simulink library "lic"  (R2021b)
settings: Solver=VariableStepAuto  StartTime=0.0  StopTime=10.0  RelTol=1e-3
undefined symbols (not defined in the file or in its folder): C_TICK_TIME_S, ENUM_LANEQUALITY_HIGH, ENUM_LANEQUALITY_MEDIUM, ENUM_LFCSTATE_DEGRADED, FALSE, KAPP_VehicleWidth_m, KLIC_C0CrossingThr_m, KLIC_C1Max4Act_rad, KLIC_C2Max4Act_rat, KLIC_C2Max4Disable_rat, KLIC_C2Max4DisableThr_s, KLIC_CalDefaultTLC_s, KLIC_CalTLCMax_s, KLIC_CalTLCMin_s, KLIC_DefaultLaneWidth_m, KLIC_Lane4ActThr_s, KLIC_LANEQUALITY_rat, KLIC_LANEQUALITYHysis_rat, KLIC_LaneWidHoldOnTime_s, KLIC_LaneWidRampFinErrThres_m, KLIC_LaneWidRampFinTimeThres_s, KLIC_LaneWidRampInFalRt_mps, KLIC_LaneWidRampInRisRt_mps, KLIC_LaneWidRampOutFalRt_mps, KLIC_LaneWidRampOutRisRt_mps, KLIC_LaneWidthLowThr_m, KLIC_LaneWidthUpThr_m, KLIC_TLCTriggerThrHysis_s, MLIC_TLCThr4LKA_s, TRUE
libraries: adcu_lib x20, simulink x14
(part 2 of 3)

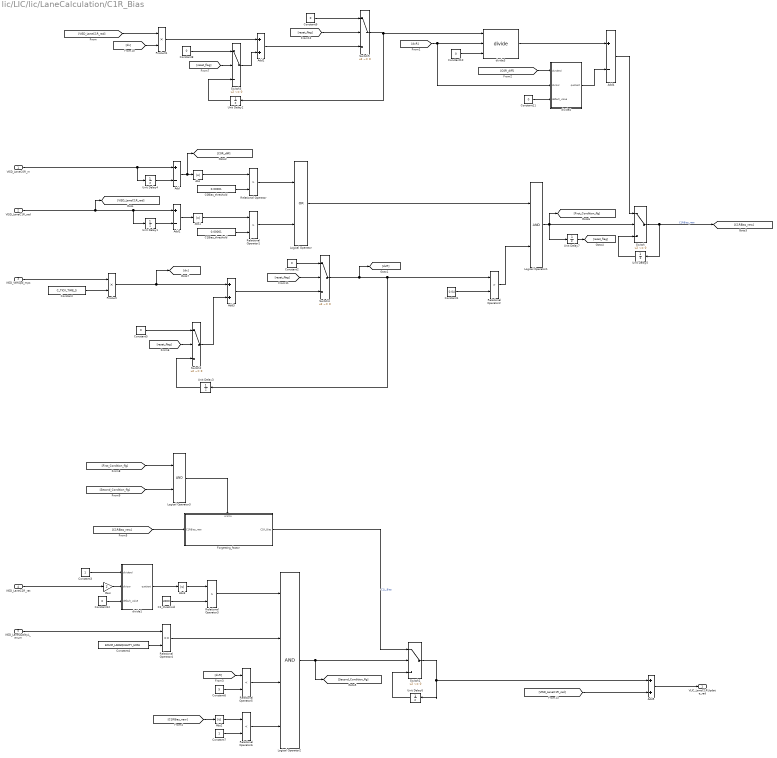
== system lic/LIC/lic/LaneCalculation/C1R_Bias ==
  VISD_LaneC0R_m : Inport
  VISD_LaneC1R_rad : Inport  Port=2
  VISD_VehSpd_mps : Inport  Port=3
  VISD_LaneC2R_rat : Inport  Port=4
  VISD_LaneQualityL_enum : Inport  Port=5
  Abs{,1..3} (4 alike) : Abs
  Add : Sum  Inputs=+-
  Add1 : Sum  Inputs=+-
  Add2 : Sum
  Add3 : Sum
  Add4 : Sum  Inputs=+-
  Add5 : Sum
  C0Bias_threshold : Constant  Value=0.00001  OutDataTypeStr=single
  C1Bias_threshold : Constant  Value=0.00001  OutDataTypeStr=single
  C2_threshold : Constant  Value=3000  OutDataTypeStr=single
  Constant : Constant  Value=C_TICK_TIME_S
  Constant1 : Constant  Value=0.04  OutDataTypeStr=single
  Constant{2,5,8..12} (7 alike) : Constant  Value=0  OutDataTypeStr=single
  Constant3 : Constant  OutDataTypeStr=single
  Constant4 : Constant  Value=ENUM_LANEQUALITY_HIGH
  Constant6 : Constant  Value=5  OutDataTypeStr=single
  Constant7 : Constant  OutDataTypeStr=single
  Forgetting_factor : Subsystem  TreatAsAtomicUnit=on
  Gain : Gain  Gain=2
  Logical Operator : Logic  Operator=OR  AllPortsSameDT=off  OutDataTypeStr=boolean
  Logical Operator1 : Logic  AllPortsSameDT=off  OutDataTypeStr=boolean
  Logical Operator2 : Logic  Inputs=4  AllPortsSameDT=off  OutDataTypeStr=boolean
  Logical Operator3 : Logic  AllPortsSameDT=off  OutDataTypeStr=boolean
  Product : Product
  Product1 : Product
  Relational Operator{,1..3} (4 alike) : RelationalOperator  Operator=>  OutDataTypeStr=boolean  RndMeth=Nearest
  Relational Operator4 : RelationalOperator  Operator===  OutDataTypeStr=boolean  RndMeth=Nearest
  Relational Operator5 : RelationalOperator  Operator=<  OutDataTypeStr=boolean  RndMeth=Nearest
  Relational Operator6 : RelationalOperator  Operator=<  OutDataTypeStr=boolean  RndMeth=Nearest
  Switch{,1..5} (6 alike) : Switch  Criteria=u2 ~= 0
  Unit Delay{1..7} (7 alike) : UnitDelay  SampleTime=-1  HasFrameUpgradeWarning=on
  divide1 : Subsystem  TreatAsAtomicUnit=on  RTWFcnName=divide_lib  RTWFileName=HCU_LIB  mask(divide){}
      mask help: Performs a division operation. If the divisor is found to be between -0.00001 and +0.00001 then a failsafe value is passed to the output.
      settings: RTWFcnNameOpts=User specified  RTWFileNameOpts=User specified
      mask Display: disp('Divide');
  divide3 : adcu_lib/divide
      settings: SourceProductName=ADAS Reusable Library
  divide4 : Subsystem  TreatAsAtomicUnit=on  RTWFcnName=divide_lib  RTWFileName=HCU_LIB  mask(divide){}
      mask help: Performs a division operation. If the divisor is found to be between -0.00001 and +0.00001 then a failsafe value is passed to the output.
      settings: RTWFcnNameOpts=User specified  RTWFileNameOpts=User specified
      mask Display: disp('Divide');
  VLIC_LaneC1RUpdate_rad : Outport
  wires:
  Add5/1 -> VLIC_LaneC1RUpdate_rad/1
  [VISD_LaneC1R_rad] -> Add5/2
  VISD_LaneC0R_m/1 -> Unit Delay4/1, Add/1
  Unit Delay4/1 -> Add/2
  VISD_LaneC1R_rad/1 -> [VISD_LaneC1R_rad], Unit Delay1/1, Add1/1
  Unit Delay1/1 -> Add1/2
  Add/1 -> [C0R_diff], Abs/1
  Add1/1 -> Abs1/1
  VISD_VehSpd_mps/1 -> Product/1
  Abs/1 -> Relational Operator/1
  C0Bias_threshold/1 -> Relational Operator/2
  Abs1/1 -> Relational Operator1/1
  C1Bias_threshold/1 -> Relational Operator1/2
  Add3/1 -> Switch4/3
  Constant1/1 -> Relational Operator2/2
  Relational Operator/1 -> Logical Operator/1
  Relational Operator1/1 -> Logical Operator/2
  Logical Operator/1 -> Logical Operator1/1
  Relational Operator2/1 -> Logical Operator1/2
  Logical Operator1/1 -> Switch/2, [First_Condition_flg], Unit Delay7/1
  [dx] -> Product1/2
  [VISD_LaneC1R_rad] -> Product1/1
  Product1/1 -> Add2/1
  Constant/1 -> Product/2
  Product/1 -> [dx], Add3/1
  [dxR] -> divide4/2(divisor), divide3/2
  divide3/1 -> Add4/1
  [C0R_diff] -> divide4/1(dividend)
  divide4/1(quotient) -> Add4/2
  Add4/1 -> Switch/1
  VISD_LaneC2R_rat/1 -> Gain/1
  divide1/1(quotient) -> Abs3/1
  C2_threshold/1 -> Relational Operator3/2
  VISD_LaneQualityL_enum/1 -> Relational Operator4/1
  Constant4/1 -> Relational Operator4/2
  Relational Operator3/1 -> Logical Operator2/1
  Relational Operator4/1 -> Logical Operator2/2
  [dxR] -> Relational Operator5/1
  Constant6/1 -> Relational Operator5/2
  Relational Operator5/1 -> Logical Operator2/3
  Relational Operator6/1 -> Logical Operator2/4
  Switch/1 -> Unit Delay5/1, [C1RBias_new]  "C1RBias_new"
  Switch1/1 -> Unit Delay6/1, Add5/1
  [C1RBias_new] -> Abs2/1
  Abs2/1 -> Relational Operator6/1
  Constant7/1 -> Relational Operator6/2
  Forgetting_factor/1(C1R_Bias) -> Switch1/1  "C1L_Bias"
  [C1RBias_new] -> Forgetting_factor/1(C1RBias_new)
  Unit Delay5/1 -> Switch/3
  Unit Delay6/1 -> Switch1/3
  Abs3/1 -> Relational Operator3/1
  Logical Operator2/1 -> [Second_Condition_flg], Switch1/2
  Switch2/1 -> Add3/2
  Constant5/1 -> Switch2/1
  [reset_flag] -> Switch2/2
  Constant8/1 -> Switch3/1
  [reset_flag] -> Switch3/2
  Switch3/1 -> Add2/2
  Unit Delay7/1 -> [reset_flag]
  Unit Delay2/1 -> Switch3/3
  Unit Delay3/1 -> Switch2/3
  [First_Condition_flg] -> Logical Operator3/1
  [Second_Condition_flg] -> Logical Operator3/2
  Logical Operator3/1 -> Forgetting_factor/Enable
  [reset_flag] -> Switch4/2
  Constant2/1 -> Switch4/1
  Switch4/1 -> [dxR], Unit Delay3/1, Relational Operator2/1
  Add2/1 -> Switch5/3
  [reset_flag] -> Switch5/2
  Constant9/1 -> Switch5/1
  Switch5/1 -> divide3/1, Unit Delay2/1
  Constant10/1 -> divide3/3
  Constant11/1 -> divide4/3(default_value)
  Constant3/1 -> divide1/1(dividend)
  Gain/1 -> divide1/2(divisor)
  Constant12/1 -> divide1/3(default_value)

== system lic/LIC/lic/LaneCalculation/GenerateLeftLane ==
  VISD_LaneC0L_m : Inport
  VLIC_EstLaneC0L_m : Inport  Port=2
  VISD_LaneC1L_rad : Inport  Port=3
  VLIC_EstLaneC1L_rad : Inport  Port=4
  VISD_LaneC2L_rat : Inport  Port=5
  VLIC_EstLaneC2L_rat : Inport  Port=6
  VISD_LaneC3L_rat : Inport  Port=7
  VLIC_EstLaneC3L_rat : Inport  Port=8
  VLIC_LeftLaneAvail_flg : Inport  Port=9
  Switch{3,12..14} (4 alike) : Switch  Criteria=u2 ~= 0
  VLIC_LaneC0L_m : Outport
  VLIC_LaneC1L_rad : Outport  Port=2
  VLIC_LaneC2L_rat : Outport  Port=3
  VLIC_LaneC3L_rat : Outport  Port=4
  wires:
  VLIC_EstLaneC0L_m/1 -> Switch3/3
  Switch12/1 -> VLIC_LaneC1L_rad/1  "VLIC_LaneC1L_rad"
  VLIC_EstLaneC1L_rad/1 -> Switch12/3
  VISD_LaneC1L_rad/1 -> Switch12/1
  Switch3/1 -> VLIC_LaneC0L_m/1  "VLIC_LaneC0L_m"
  Switch13/1 -> VLIC_LaneC2L_rat/1  "VLIC_LaneC2L_rat"
  VLIC_EstLaneC2L_rat/1 -> Switch13/3
  VISD_LaneC2L_rat/1 -> Switch13/1
  VLIC_LeftLaneAvail_flg/1 -> Switch14/2, Switch13/2, Switch12/2, Switch3/2
  VLIC_EstLaneC3L_rat/1 -> Switch14/3
  VISD_LaneC3L_rat/1 -> Switch14/1
  VISD_LaneC0L_m/1 -> Switch3/1
  Switch14/1 -> VLIC_LaneC3L_rat/1  "VLIC_LaneC3L_rat"

== system lic/LIC/lic/LaneCalculation/GenerateRightLane ==
  VISD_LaneC0R_m : Inport
  VLIC_EstLaneC0R_m : Inport  Port=2
  VISD_LaneC1R_rad : Inport  Port=3
  VLIC_EstLaneC1R_rad : Inport  Port=4
  VISD_LaneC2R_rat : Inport  Port=5
  VLIC_EstLaneC2R_rat : Inport  Port=6
  VISD_LaneC3R_rat : Inport  Port=7
  VLIC_EstLaneC3R_rat : Inport  Port=8
  VLIC_RightLaneAvail_flg : Inport  Port=9
  Switch{3,12..14} (4 alike) : Switch  Criteria=u2 ~= 0
  VLIC_LaneC0R_m : Outport
  VLIC_LaneC1R_rad : Outport  Port=2
  VLIC_LaneC2R_rat : Outport  Port=3
  VLIC_LaneC3R_rat : Outport  Port=4
  wires:
  VISD_LaneC0R_m/1 -> Switch3/1
  VISD_LaneC3R_rat/1 -> Switch14/1
  VLIC_EstLaneC3R_rat/1 -> Switch14/3
  Switch14/1 -> VLIC_LaneC3R_rat/1  "VLIC_LaneC3R_rat"
  VLIC_RightLaneAvail_flg/1 -> Switch3/2, Switch12/2, Switch13/2, Switch14/2
  VISD_LaneC2R_rat/1 -> Switch13/1
  VLIC_EstLaneC2R_rat/1 -> Switch13/3
  Switch13/1 -> VLIC_LaneC2R_rat/1  "VLIC_LaneC2R_rat"
  Switch3/1 -> VLIC_LaneC0R_m/1  "VLIC_LaneC0R_m"
  VISD_LaneC1R_rad/1 -> Switch12/1
  VLIC_EstLaneC1R_rad/1 -> Switch12/3
  Switch12/1 -> VLIC_LaneC1R_rad/1  "VLIC_LaneC1R_rad"
  VLIC_EstLaneC0R_m/1 -> Switch3/3

== system lic/LIC/lic/LaneCalculation/LR_Available ==
  VISD_LaneC0L_m : Inport
  VISD_LaneC0R_m : Inport  Port=2
  VISD_LaneC1L_rad : Inport  Port=3
  VISD_LaneC1R_rad : Inport  Port=4
  VISD_LaneC2L_rat : Inport  Port=5
  VISD_LaneC2R_rat : Inport  Port=6
  VISD_LaneC3L_rat : Inport  Port=7
  VISD_LaneC3R_rat : Inport  Port=8
  Enable : EnablePort  StatesWhenEnabling=reset
  Add{,1..3} (4 alike) : Sum
  Gain{,1..3} (4 alike) : Gain  Gain=0.5
  VLIC_RLCenterLineC0_m : Outport
  VLIC_RLCenterLineC1_rad : Outport  Port=2
  VLIC_RLCenterLineC2_rat : Outport  Port=3
  VLIC_RLCenterLineC3_rat : Outport  Port=4
  wires:
  VISD_LaneC0L_m/1 -> Add/1
  VISD_LaneC0R_m/1 -> Add/2
  Add/1 -> Gain/1
  Gain/1 -> VLIC_RLCenterLineC0_m/1  "VLIC_RLCenterLineC0_m"
  VISD_LaneC1L_rad/1 -> Add1/1
  VISD_LaneC1R_rad/1 -> Add1/2
  Add1/1 -> Gain1/1
  Add2/1 -> Gain2/1
  Gain1/1 -> VLIC_RLCenterLineC1_rad/1  "VLIC_RLCenterLineC1_rad"
  VISD_LaneC2L_rat/1 -> Add2/1
  VISD_LaneC2R_rat/1 -> Add2/2
  Gain2/1 -> VLIC_RLCenterLineC2_rat/1  "VLIC_RLCenterLineC2_rat"
  Add3/1 -> Gain3/1
  VISD_LaneC3L_rat/1 -> Add3/1
  VISD_LaneC3R_rat/1 -> Add3/2
  Gain3/1 -> VLIC_RLCenterLineC3_rat/1  "VLIC_RLCenterLineC3_rat"

== system lic/LIC/lic/LaneCalculation/LR_NotAvailable ==
  VLIC_EstLaneC0L_m : Inport
  VLIC_EstLaneC0R_m : Inport  Port=2
  VLIC_EstLaneC1L_rad : Inport  Port=3
  VLIC_EstLaneC1R_rad : Inport  Port=4
  VLIC_EstLaneC2L_rat : Inport  Port=5
  VLIC_EstLaneC2R_rat : Inport  Port=6
  VLIC_EstLaneC3L_rat : Inport  Port=7
  VLIC_EstLaneC3R_rat : Inport  Port=8
  Enable : EnablePort  StatesWhenEnabling=reset
  Add{,1..3} (4 alike) : Sum
  Gain{,1..3} (4 alike) : Gain  Gain=0.5
  VLIC_EstCenterLineC0_m : Outport
  VLIC_EstCenterLineC1_rad : Outport  Port=2
  VLIC_EstCenterLineC2_rat : Outport  Port=3
  VLIC_EstCenterLineC3_rat : Outport  Port=4
  wires:
  VLIC_EstLaneC0L_m/1 -> Add/1
  VLIC_EstLaneC0R_m/1 -> Add/2
  Add/1 -> Gain/1
  Gain/1 -> VLIC_EstCenterLineC0_m/1  "VLIC_EstCenterLineC0_m"
  VLIC_EstLaneC1L_rad/1 -> Add1/1
  VLIC_EstLaneC1R_rad/1 -> Add1/2
  Add1/1 -> Gain1/1
  Add2/1 -> Gain2/1
  Gain1/1 -> VLIC_EstCenterLineC1_rad/1  "VLIC_EstCenterLineC1_rad"
  VLIC_EstLaneC2L_rat/1 -> Add2/1
  VLIC_EstLaneC2R_rat/1 -> Add2/2
  Gain2/1 -> VLIC_EstCenterLineC2_rat/1  "VLIC_EstCenterLineC2_rat"
  Add3/1 -> Gain3/1
  VLIC_EstLaneC3L_rat/1 -> Add3/1
  VLIC_EstLaneC3R_rat/1 -> Add3/2
  Gain3/1 -> VLIC_EstCenterLineC3_rat/1  "VLIC_EstCenterLineC3_rat"

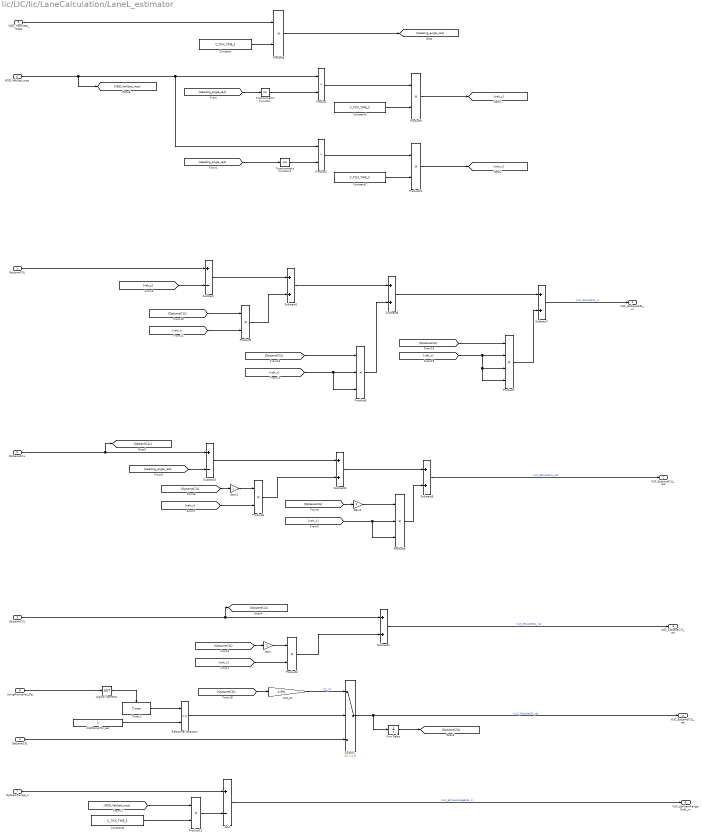
== system lic/LIC/lic/LaneCalculation/LaneL_estimator ==
  OptLaneC0L : Inport
  OptLaneC1L : Inport  Port=2
  OptLaneC2L : Inport  Port=3
  OptLaneC3L : Inport  Port=4
  VISD_YawRate_radps : Inport  Port=5
  VISD_VehSpd_mps : Inport  Port=6
  OptViewRange_L : Inport  Port=7
  UsingRawLaneL_flg : Inport  Port=8
  Add : Sum  Inputs=+-
  C3LRampThr_sec : Constant  OutDataTypeStr=single
  C3L_FF : Gain  Gain=0.994
  Constant{,1..2,4} (4 alike) : Constant  Value=C_TICK_TIME_S
  Gain : Gain  Gain=3
  Gain1 : Gain  Gain=2
  Gain2 : Gain  Gain=3
  Logical Operator : Logic  Operator=NOT  AllPortsSameDT=off  OutDataTypeStr=boolean
  Product{,1..3,5,8..10,12} (9 alike) : Product
  Product4 : Product  Inputs=3
  Product6 : Product  Inputs=3
  Product7 : Product  Inputs=4
  Relational Operator : RelationalOperator  OutDataTypeStr=boolean  RndMeth=Nearest
  Subtract : Sum  Inputs=+-
  Subtract{1..2,4..7} (6 alike) : Sum
  Subtract3 : Sum  Inputs=+-
  Switch2 : Switch  Criteria=u2 ~= 0
  Timer1 : adcu_lib/Timer  SystemSampleTime=-1  VariantActivationTime=update diagram  Latency=0  AutoFrameSizeCalculation=off
      settings: SourceProductName=ADAS Reusable Library
  Trigonometric Function : Trigonometry
  Trigonometric Function1 : Trigonometry  Operator=cos
  Unit Delay : UnitDelay  SampleTime=-1  HasFrameUpgradeWarning=on
  VLIC_EstLaneC0L_m : Outport
  VLIC_EstLaneC1L_rad : Outport  Port=2
  VLIC_EstLaneC2L_rat : Outport  Port=3
  VLIC_EstLaneC3L_rat : Outport  Port=4
  VLIC_EstViewRangeEndL_m : Outport  Port=5
  wires:
  VISD_VehSpd_mps/1 -> [VISD_VehSpd_mps], Product1/1, Product/1
  [Heading_angle_rad] -> Trigonometric Function/1
  Trigonometric Function/1 -> Product/2
  Product9/1 -> [veh_y]
  [Heading_angle_rad] -> Trigonometric Function1/1
  Trigonometric Function1/1 -> Product1/2
  Product10/1 -> [veh_x]
  OptLaneC0L/1 -> Subtract/1
  [veh_y] -> Subtract/2
  Subtract/1 -> Subtract1/1
  OptLaneC2L/1 -> [OptLaneC2L], Subtract2/1
  Product2/1 -> Subtract2/2
  [OptLaneC3L] -> Gain/1
  Gain/1 -> Product2/1
  [veh_x] -> Product2/2
  Subtract2/1 -> VLIC_EstLaneC2L_rat/1  "VLIC_EstLaneC2L_rat"
  OptLaneC1L/1 -> [OptLaneC1L], Subtract3/1
  [Heading_angle_rad] -> Subtract3/2
  Subtract3/1 -> Subtract4/1
  [OptLaneC2L] -> Gain1/1
  Gain1/1 -> Product3/1
  [veh_x] -> Product3/2
  Product3/1 -> Subtract4/2
  Subtract4/1 -> Subtract5/1
  [OptLaneC3L] -> Gain2/1
  Gain2/1 -> Product4/1
  [veh_x] -> Product4/3, Product4/2
  Product4/1 -> Subtract5/2
  Subtract5/1 -> VLIC_EstLaneC1L_rad/1  "VLIC_EstLaneC1L_rad"
  [OptLaneC1L] -> Product5/1
  [veh_x] -> Product5/2
  Product5/1 -> Subtract1/2
  Subtract1/1 -> Subtract6/1
  [OptLaneC2L] -> Product6/1
  [veh_x] -> Product6/2, Product6/3
  Product6/1 -> Subtract6/2
  Subtract6/1 -> Subtract7/1
  [OptLaneC3L] -> Product7/1
  [veh_x] -> Product7/2, Product7/4, Product7/3
  Product7/1 -> Subtract7/2
  Subtract7/1 -> VLIC_EstLaneC0L_m/1  "VLIC_EstLaneC0L_m"
  Constant/1 -> Product8/2
  Constant1/1 -> Product9/2
  Product/1 -> Product9/1
  Constant2/1 -> Product10/2
  Product1/1 -> Product10/1
  VISD_YawRate_radps/1 -> Product8/1
  OptViewRange_L/1 -> Add/1
  [VISD_VehSpd_mps] -> Product12/1
  Product12/1 -> Add/2
  Add/1 -> VLIC_EstViewRangeEndL_m/1  "VLIC_EstViewRangeEndL_m"
  Constant4/1 -> Product12/2
  UsingRawLaneL_flg/1 -> Logical Operator/1
  Timer1/1 -> Relational Operator/1
  C3LRampThr_sec/1 -> Relational Operator/2
  Relational Operator/1 -> Switch2/2
  OptLaneC3L/1 -> Switch2/3
  Switch2/1 -> Unit Delay/1, VLIC_EstLaneC3L_rat/1  "VLIC_EstLaneC3L_rat"
  [OptLaneC3L] -> C3L_FF/1
  C3L_FF/1 -> Switch2/1  "C3L_FF"
  Logical Operator/1 -> Timer1/Enable
  Unit Delay/1 -> [OptLaneC3L]
  Product8/1 -> [Heading_angle_rad]

== system lic/LIC/lic/LaneCalculation/LaneProcess ==
  VINP_LnMk1Side_enum : Inport
  VINP_LnMk2Side_enum : Inport  Port=2
  VINP_Ln1C0_m : Inport  Port=3
  VINP_Ln1C1_rad : Inport  Port=4
  VINP_Ln1C2_1pm : Inport  Port=5
  VINP_Ln1C3_1pmm : Inport  Port=6
  VINP_Ln2C0_m : Inport  Port=7
  VINP_Ln2C1_rad : Inport  Port=8
  VINP_Ln2C2_1pm : Inport  Port=9
  VINP_Ln2C3_1pmm : Inport  Port=10
  VINP_LnMk1Cnfdnce_rad : Inport  Port=11
  VINP_LnMk2Cnfdnce_rad : Inport  Port=12
  VINP_LnMk1StartVR_m : Inport  Port=13
  VINP_LnMk1EndVR_m : Inport  Port=14
  VINP_LnMk2StartVR_m : Inport  Port=15
  VINP_LnMk2EndVR_m : Inport  Port=16
  Chart : Stateflow chart  TreatAsAtomicUnit=on
  VLIC_HLC0L_m : Outport
  VLIC_HLC1L_rad : Outport  Port=2
  VLIC_HLC2L_1pm : Outport  Port=3
  VLIC_HLC3L_1pmm : Outport  Port=4
  VLIC_HLC0R_m : Outport  Port=5
  VLIC_HLC1R_rad : Outport  Port=6
  VLIC_HLC2R_1pm : Outport  Port=7
  VLIC_HLC3R_1pmm : Outport  Port=8
  VLIC_HLViewRangeL_m : Outport  Port=9
  VLIC_HLViewRangeR_m : Outport  Port=10
  VLIC_HLQualityL_rat : Outport  Port=11
  VLIC_HLQualityR_rat : Outport  Port=12
  wires:
  VINP_LnMk1Side_enum/1 -> Chart/1(VINP_LnMk1Side_enum)
  VINP_LnMk2Side_enum/1 -> Chart/2(VINP_LnMk2Side_enum)
  VINP_Ln1C0_m/1 -> Chart/3(VINP_Ln1C0_m)
  VINP_Ln1C1_rad/1 -> Chart/4(VINP_Ln1C1_rad)
  VINP_Ln1C2_1pm/1 -> Chart/5(VINP_Ln1C2_1pm)
  VINP_Ln1C3_1pmm/1 -> Chart/6(VINP_Ln1C3_1pmm)
  VINP_Ln2C0_m/1 -> Chart/7(VINP_Ln2C0_m)
  VINP_Ln2C1_rad/1 -> Chart/8(VINP_Ln2C1_rad)
  VINP_Ln2C2_1pm/1 -> Chart/9(VINP_Ln2C2_1pm)
  VINP_Ln2C3_1pmm/1 -> Chart/10(VINP_Ln2C3_1pmm)
  Chart/2(VLIC_HLC1L_rad) -> VLIC_HLC1L_rad/1
  Chart/1(VLIC_HLC0L_m) -> VLIC_HLC0L_m/1
  Chart/3(VLIC_HLC2L_1pm) -> VLIC_HLC2L_1pm/1
  Chart/4(VLIC_HLC3L_1pmm) -> VLIC_HLC3L_1pmm/1
  VINP_LnMk1Cnfdnce_rad/1 -> Chart/11(VINP_LnMk1Cnfdnce_rad)
  VINP_LnMk2Cnfdnce_rad/1 -> Chart/12(VINP_LnMk2Cnfdnce_rad)
  VINP_LnMk1StartVR_m/1 -> Chart/13(VINP_LnMk1StartVR_m)
  VINP_LnMk1EndVR_m/1 -> Chart/14(VINP_LnMk1EndVR_m)
  VINP_LnMk2StartVR_m/1 -> Chart/15(VINP_LnMk2StartVR_m)
  VINP_LnMk2EndVR_m/1 -> Chart/16(VINP_LnMk2EndVR_m)
  Chart/5(VLIC_HLC0R_m) -> VLIC_HLC0R_m/1
  Chart/6(VLIC_HLC1R_rad) -> VLIC_HLC1R_rad/1
  Chart/7(VLIC_HLC2R_1pm) -> VLIC_HLC2R_1pm/1
  Chart/8(VLIC_HLC3R_1pmm) -> VLIC_HLC3R_1pmm/1
  Chart/9(VLIC_HLViewRangeL_m) -> VLIC_HLViewRangeL_m/1
  Chart/10(VLIC_HLViewRangeR_m) -> VLIC_HLViewRangeR_m/1
  Chart/11(VLIC_HLQualityL_rat) -> VLIC_HLQualityL_rat/1
  Chart/12(VLIC_HLQualityR_rat) -> VLIC_HLQualityR_rat/1

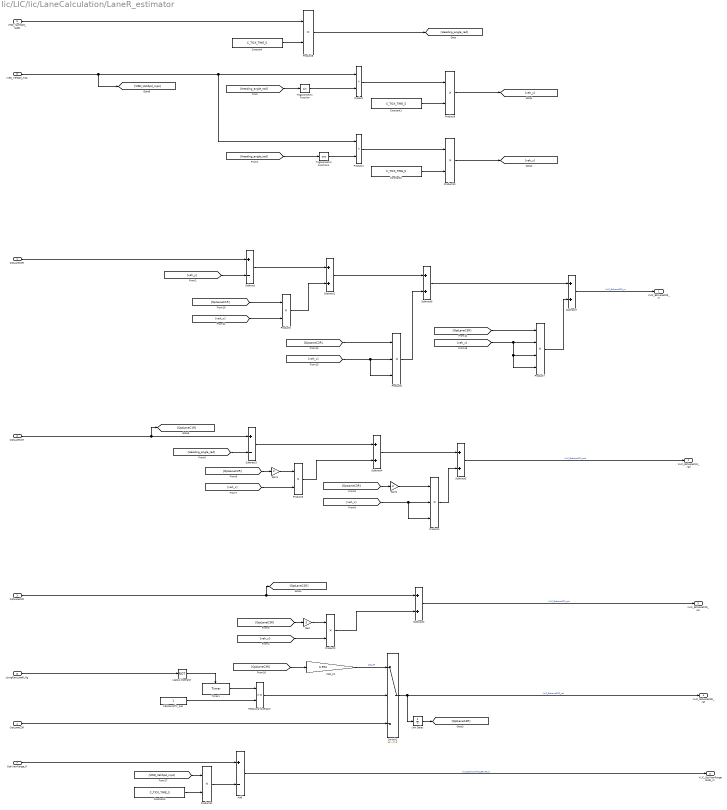
== system lic/LIC/lic/LaneCalculation/LaneR_estimator ==
  OptLaneC0R : Inport
  OptLaneC1R : Inport  Port=2
  OptLaneC2R : Inport  Port=3
  OptLaneC3R : Inport  Port=4
  VISD_YawRate_radps : Inport  Port=5
  VISD_VehSpd_mps : Inport  Port=6
  OptViewRange_R : Inport  Port=7
  UsingRawLaneR_flg : Inport  Port=8
  Add : Sum  Inputs=+-
  C3LRampThr_sec : Constant  OutDataTypeStr=single
  C3R_FF : Gain  Gain=0.994
  Constant{,1..2,4} (4 alike) : Constant  Value=C_TICK_TIME_S
  Gain : Gain  Gain=3
  Gain1 : Gain  Gain=2
  Gain2 : Gain  Gain=3
  Logical Operator : Logic  Operator=NOT  AllPortsSameDT=off  OutDataTypeStr=boolean
  Product{,1..3,5,8..10,12} (9 alike) : Product
  Product4 : Product  Inputs=3
  Product6 : Product  Inputs=3
  Product7 : Product  Inputs=4
  Relational Operator : RelationalOperator  OutDataTypeStr=boolean  RndMeth=Nearest
  Subtract : Sum  Inputs=+-
  Subtract{1..2,4..7} (6 alike) : Sum
  Subtract3 : Sum  Inputs=+-
  Switch2 : Switch  Criteria=u2 ~= 0
  Timer1 : adcu_lib/Timer  SystemSampleTime=-1  VariantActivationTime=update diagram  Latency=0  AutoFrameSizeCalculation=off
      settings: SourceProductName=ADAS Reusable Library
  Trigonometric Function : Trigonometry
  Trigonometric Function1 : Trigonometry  Operator=cos
  Unit Delay : UnitDelay  SampleTime=-1  HasFrameUpgradeWarning=on
  VLIC_EstLaneC0R_m : Outport
  VLIC_EstLaneC1R_rad : Outport  Port=2
  VLIC_EstLaneC2R_rat : Outport  Port=3
  VLIC_EstLaneC3R_rat : Outport  Port=4
  VLIC_EstViewRangeEndR_m : Outport  Port=5
  wires:
  Add/1 -> VLIC_EstViewRangeEndR_m/1  "VLIC_EstViewRangeEndR_m"
  Product12/1 -> Add/2
  Constant4/1 -> Product12/2
  [VISD_VehSpd_mps] -> Product12/1
  OptViewRange_R/1 -> Add/1
  Product8/1 -> [Heading_angle_rad]
  VISD_YawRate_radps/1 -> Product8/1
  Product1/1 -> Product10/1
  Constant2/1 -> Product10/2
  Product/1 -> Product9/1
  Constant1/1 -> Product9/2
  Constant/1 -> Product8/2
  Subtract7/1 -> VLIC_EstLaneC0R_m/1  "VLIC_EstLaneC0R_m"
  Product7/1 -> Subtract7/2
  [veh_x] -> Product7/3, Product7/4, Product7/2
  [OptLaneC3R] -> Product7/1
  Subtract6/1 -> Subtract7/1
  Product6/1 -> Subtract6/2
  [veh_x] -> Product6/3, Product6/2
  [OptLaneC2R] -> Product6/1
  Subtract1/1 -> Subtract6/1
  Product5/1 -> Subtract1/2
  [veh_x] -> Product5/2
  [OptLaneC1R] -> Product5/1
  Subtract5/1 -> VLIC_EstLaneC1R_rad/1  "VLIC_EstLaneC1R_rad"
  Product4/1 -> Subtract5/2
  [veh_x] -> Product4/2, Product4/3
  Gain2/1 -> Product4/1
  [OptLaneC3R] -> Gain2/1
  Subtract4/1 -> Subtract5/1
  Product3/1 -> Subtract4/2
  [veh_x] -> Product3/2
  Gain1/1 -> Product3/1
  [OptLaneC2R] -> Gain1/1
  Subtract3/1 -> Subtract4/1
  [Heading_angle_rad] -> Subtract3/2
  OptLaneC1R/1 -> Subtract3/1, [OptLaneC1R]
  Subtract2/1 -> VLIC_EstLaneC2R_rat/1  "VLIC_EstLaneC2R_rat"
  [veh_x] -> Product2/2
  Gain/1 -> Product2/1
  [OptLaneC3R] -> Gain/1
  Product2/1 -> Subtract2/2
  OptLaneC2R/1 -> Subtract2/1, [OptLaneC2R]
  Subtract/1 -> Subtract1/1
  [veh_y] -> Subtract/2
  OptLaneC0R/1 -> Subtract/1
  Product10/1 -> [veh_x]
  Trigonometric Function1/1 -> Product1/2
  [Heading_angle_rad] -> Trigonometric Function1/1
  Product9/1 -> [veh_y]
  Trigonometric Function/1 -> Product/2
  [Heading_angle_rad] -> Trigonometric Function/1
  VISD_VehSpd_mps/1 -> Product/1, Product1/1, [VISD_VehSpd_mps]
  UsingRawLaneR_flg/1 -> Logical Operator/1
  Timer1/1 -> Relational Operator/1
  C3LRampThr_sec/1 -> Relational Operator/2
  Relational Operator/1 -> Switch2/2
  Switch2/1 -> Unit Delay/1, VLIC_EstLaneC3R_rat/1  "VLIC_EstLaneC3R_rat"
  [OptLaneC3R] -> C3R_FF/1
  C3R_FF/1 -> Switch2/1  "C3R_FF"
  OptLaneC3R/1 -> Switch2/3
  Logical Operator/1 -> Timer1/Enable
  Unit Delay/1 -> [OptLaneC3R]

== system lic/LIC/lic/LaneCalculation/LaneResidual_Calculation ==
  VLIC_EstViewRangeEndL_m : Inport
  VISD_VehSpd_mps : Inport  Port=2
  VLIC_EstViewRangeEndR_m : Inport  Port=3
  Constant6 : Constant  Value=3  OutDataTypeStr=single
  Constant7 : Constant  Value=3  OutDataTypeStr=single
  Saturation1 : Saturate  UpperLimit=3  LowerLimit=0
      settings: AttributesFormatString=upper = %<UpperLimit>\nlower = %<LowerLimit>
  Saturation2 : Saturate  UpperLimit=3  LowerLimit=0
      settings: AttributesFormatString=upper = %<UpperLimit>\nlower = %<LowerLimit>
  divide1 : Subsystem  TreatAsAtomicUnit=on  RTWFcnName=divide_lib  RTWFileName=HCU_LIB  mask(divide){}
      mask help: Performs a division operation. If the divisor is found to be between -0.00001 and +0.00001 then a failsafe value is passed to the output.
      settings: RTWFcnNameOpts=User specified  RTWFileNameOpts=User specified
      mask Display: disp('Divide');
  divide3 : Subsystem  TreatAsAtomicUnit=on  RTWFcnName=divide_lib  RTWFileName=HCU_LIB  mask(divide){}
      mask help: Performs a division operation. If the divisor is found to be between -0.00001 and +0.00001 then a failsafe value is passed to the output.
      settings: RTWFcnNameOpts=User specified  RTWFileNameOpts=User specified
      mask Display: disp('Divide');
  VLIC_ResidualLaneL_s : Outport
  VLIC_ResidualLaneR_s : Outport  Port=2
  wires:
  divide3/1(quotient) -> Saturation1/1
  VLIC_EstViewRangeEndL_m/1 -> divide3/1(dividend)
  Constant6/1 -> divide3/3(default_value)
  VLIC_EstViewRangeEndR_m/1 -> divide1/1(dividend)
  VISD_VehSpd_mps/1 -> divide1/2(divisor), divide3/2(divisor)
  Constant7/1 -> divide1/3(default_value)
  divide1/1(quotient) -> Saturation2/1
  Saturation1/1 -> VLIC_ResidualLaneL_s/1  "VLIC_ResidualLaneL_s"
  Saturation2/1 -> VLIC_ResidualLaneR_s/1  "VLIC_ResidualLaneR_s"

== system lic/LIC/lic/LaneCalculation/LaneWidth ==
  VLIC_LeftLaneAvail_flg : Inport
  VLIC_RightLaneAvail_flg : Inport  Port=2
  VLIC_LaneC0L_m : Inport  Port=3
  VLIC_LaneC0R_m : Inport  Port=4
  Add : Sum  Inputs=+-
  Delay : Delay  DelayLength=1  InitialCondition=KLIC_DefaultLaneWidth_m
  KLIC_DefaultLaneWidth_m : Constant  Value=KLIC_DefaultLaneWidth_m
  KLIC_LaneWidHoldOnTime_s : Constant  Value=KLIC_LaneWidHoldOnTime_s
  KLIC_LaneWidRampFinErrThres_m : Constant  Value=KLIC_LaneWidRampFinErrThres_m
  KLIC_LaneWidRampFinTimeThres_s : Constant  Value=KLIC_LaneWidRampFinTimeThres_s
  KLIC_LaneWidRampInFalRt_mps : Constant  Value=KLIC_LaneWidRampInFalRt_mps
  KLIC_LaneWidRampInRisRt_mps : Constant  Value=KLIC_LaneWidRampInRisRt_mps
  KLIC_LaneWidRampOutFalRt_mps : Constant  Value=KLIC_LaneWidRampOutFalRt_mps
  KLIC_LaneWidRampOutRisRt_mps : Constant  Value=KLIC_LaneWidRampOutRisRt_mps
  Logical Operator : Logic  Operator=OR  AllPortsSameDT=off  OutDataTypeStr=boolean
  Logical Operator1 : Logic  Operator=NOT  AllPortsSameDT=off  OutDataTypeStr=boolean
  Logical Operator2 : Logic  Operator=NOT  AllPortsSameDT=off  OutDataTypeStr=boolean
  RampInRampOut2 : Subsystem  TreatAsAtomicUnit=on  RTWFcnName=rampinrampout_lib  RTWFileName=HCU_LIB
      settings: RTWFcnNameOpts=User specified  RTWFileNameOpts=User specified
  Relational Operator2 : RelationalOperator  OutDataTypeStr=boolean  RndMeth=Nearest
  Switch2 : Switch  Criteria=u2 ~= 0
  Timer2 : Subsystem  TreatAsAtomicUnit=on  RTWFcnName=timer_lib  RTWFileName=HCU_LIB
      settings: RTWFcnNameOpts=User specified  RTWFileNameOpts=User specified
  VLIC_LaneWidth_m : Outport
  wires:
  VLIC_LaneC0R_m/1 -> Add/2
  Add/1 -> Switch2/3
  VLIC_LaneC0L_m/1 -> Add/1
  Logical Operator2/1 -> Logical Operator/2
  Logical Operator1/1 -> Logical Operator/1
  Switch2/1 -> RampInRampOut2/1(Data_Input)
  Delay/1 -> Switch2/1
  KLIC_DefaultLaneWidth_m/1 -> RampInRampOut2/2(RampIn_Target)
  Logical Operator/1 -> Timer2/Enable, Switch2/2
  KLIC_LaneWidRampInRisRt_mps/1 -> RampInRampOut2/4(RampIn_RisingRate)
  KLIC_LaneWidRampInFalRt_mps/1 -> RampInRampOut2/5(RampInFallingRate)
  KLIC_LaneWidRampOutFalRt_mps/1 -> RampInRampOut2/7(RampOutFallingRate)
  KLIC_LaneWidRampOutRisRt_mps/1 -> RampInRampOut2/6(RampOut_RisingRate)
  KLIC_LaneWidRampFinErrThres_m/1 -> RampInRampOut2/8(RampOutFinish_ErrThres)
  KLIC_LaneWidRampFinTimeThres_s/1 -> RampInRampOut2/9(RampOutFinish_TimeThres)
  RampInRampOut2/1(Data_Output) -> Delay/1, VLIC_LaneWidth_m/1  "VLIC_LaneWidth_m"
  Relational Operator2/1 -> RampInRampOut2/3(Ramp_Switch)
  Timer2/1(Timer (sec)) -> Relational Operator2/1
  KLIC_LaneWidHoldOnTime_s/1 -> Relational Operator2/2
  VLIC_LeftLaneAvail_flg/1 -> Logical Operator1/1
  VLIC_RightLaneAvail_flg/1 -> Logical Operator2/1

== system lic/LIC/lic/LaneCalculation/OnlyL_Available ==
  VLIC_LaneWidth_m : Inport
  VISD_LaneC0L_m : Inport  Port=2
  VISD_LaneC1L_rad : Inport  Port=3
  VISD_LaneC2L_rat : Inport  Port=4
  VISD_LaneC3L_rat : Inport  Port=5
  Enable : EnablePort  StatesWhenEnabling=reset
  Add : Sum  Inputs=-+
  Data Type Conversion : DataTypeConversion  OutDataTypeStr=single
  Data Type Conversion1 : DataTypeConversion  OutDataTypeStr=single
  Data Type Conversion2 : DataTypeConversion  OutDataTypeStr=single
  Gain : Gain  Gain=0.5
  VLIC_LCenterLineC0_m : Outport
  VLIC_LCenterLineC1_rad : Outport  Port=2
  VLIC_LCenterLineC2_rat : Outport  Port=3
  VLIC_LCenterLineC3_rat : Outport  Port=4
  wires:
  VISD_LaneC1L_rad/1 -> Data Type Conversion/1
  VLIC_LaneWidth_m/1 -> Gain/1
  VISD_LaneC0L_m/1 -> Add/2
  VISD_LaneC2L_rat/1 -> Data Type Conversion1/1
  VISD_LaneC3L_rat/1 -> Data Type Conversion2/1
  Add/1 -> VLIC_LCenterLineC0_m/1  "VLIC_LCenterLineC0_m"
  Data Type Conversion1/1 -> VLIC_LCenterLineC2_rat/1  "VLIC_LCenterLineC2_rat"
  Data Type Conversion2/1 -> VLIC_LCenterLineC3_rat/1  "VLIC_LCenterLineC3_rat"
  Data Type Conversion/1 -> VLIC_LCenterLineC1_rad/1  "VLIC_LCenterLineC1_rad"
  Gain/1 -> Add/1

== system lic/LIC/lic/LaneCalculation/OnlyR_Available ==
  VLIC_LaneWidth_m : Inport
  VISD_LaneC0R_m : Inport  Port=2
  VISD_LaneC1R_rad : Inport  Port=3
  VISD_LaneC2R_rat : Inport  Port=4
  VISD_LaneC3R_rat : Inport  Port=5
  Enable : EnablePort  StatesWhenEnabling=reset
  Add1 : Sum
  Data Type Conversion : DataTypeConversion  OutDataTypeStr=single
  Data Type Conversion1 : DataTypeConversion  OutDataTypeStr=single
  Data Type Conversion2 : DataTypeConversion  OutDataTypeStr=single
  Gain : Gain  Gain=0.5
  VLIC_RCenterLineC0_m : Outport
  VLIC_RCenterLineC1_rad : Outport  Port=2
  VLIC_RCenterLineC2_rat : Outport  Port=3
  VLIC_RCenterLineC3_rat : Outport  Port=4
  wires:
  VISD_LaneC3R_rat/1 -> Data Type Conversion2/1
  VISD_LaneC2R_rat/1 -> Data Type Conversion1/1
  VISD_LaneC0R_m/1 -> Add1/2
  VLIC_LaneWidth_m/1 -> Gain/1
  VISD_LaneC1R_rad/1 -> Data Type Conversion/1
  Gain/1 -> Add1/1
  Add1/1 -> VLIC_RCenterLineC0_m/1  "VLIC_RCenterLineC0_m"
  Data Type Conversion/1 -> VLIC_RCenterLineC1_rad/1  "VLIC_RCenterLineC1_rad"
  Data Type Conversion1/1 -> VLIC_RCenterLineC2_rat/1  "VLIC_RCenterLineC2_rat"
  Data Type Conversion2/1 -> VLIC_RCenterLineC3_rat/1  "VLIC_RCenterLineC3_rat"

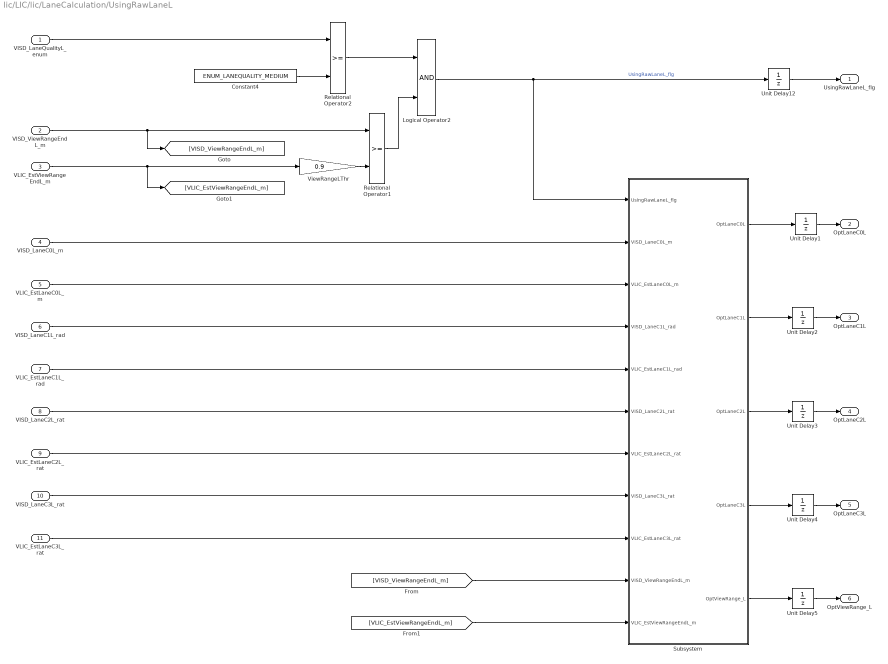
== system lic/LIC/lic/LaneCalculation/UsingRawLaneL ==
  VISD_LaneQualityL_enum : Inport
  VISD_ViewRangeEndL_m : Inport  Port=2
  VLIC_EstViewRangeEndL_m : Inport  Port=3
  VISD_LaneC0L_m : Inport  Port=4
  VLIC_EstLaneC0L_m : Inport  Port=5
  VISD_LaneC1L_rad : Inport  Port=6
  VLIC_EstLaneC1L_rad : Inport  Port=7
  VISD_LaneC2L_rat : Inport  Port=8
  VLIC_EstLaneC2L_rat : Inport  Port=9
  VISD_LaneC3L_rat : Inport  Port=10
  VLIC_EstLaneC3L_rat : Inport  Port=11
  Constant4 : Constant  Value=ENUM_LANEQUALITY_MEDIUM
  Logical Operator2 : Logic  AllPortsSameDT=off  OutDataTypeStr=boolean
  Relational Operator1 : RelationalOperator  OutDataTypeStr=boolean  RndMeth=Nearest
  Relational Operator2 : RelationalOperator  OutDataTypeStr=boolean  RndMeth=Nearest
  Subsystem : Subsystem
  Unit Delay{1..5,12} (6 alike) : UnitDelay  SampleTime=-1  HasFrameUpgradeWarning=on
  ViewRangeLThr : Gain  Gain=0.9
  UsingRawLaneL_flg : Outport
  OptLaneC0L : Outport  Port=2
  OptLaneC1L : Outport  Port=3
  OptLaneC2L : Outport  Port=4
  OptLaneC3L : Outport  Port=5
  OptViewRange_L : Outport  Port=6
  wires:
  Unit Delay5/1 -> OptViewRange_L/1
  Unit Delay4/1 -> OptLaneC3L/1
  Unit Delay3/1 -> OptLaneC2L/1
  Unit Delay2/1 -> OptLaneC1L/1
  Unit Delay1/1 -> OptLaneC0L/1
  Unit Delay12/1 -> UsingRawLaneL_flg/1
  Relational Operator1/1 -> Logical Operator2/2
  ViewRangeLThr/1 -> Relational Operator1/2
  VLIC_EstViewRangeEndL_m/1 -> [VLIC_EstViewRangeEndL_m], ViewRangeLThr/1
  VISD_ViewRangeEndL_m/1 -> [VISD_ViewRangeEndL_m], Relational Operator1/1
  Relational Operator2/1 -> Logical Operator2/1
  Constant4/1 -> Relational Operator2/2
  VISD_LaneQualityL_enum/1 -> Relational Operator2/1
  Logical Operator2/1 -> Subsystem/1(UsingRawLaneL_flg), Unit Delay12/1  "UsingRawLaneL_flg"
  VISD_LaneC0L_m/1 -> Subsystem/2(VISD_LaneC0L_m)
  VLIC_EstLaneC0L_m/1 -> Subsystem/3(VLIC_EstLaneC0L_m)
  VISD_LaneC1L_rad/1 -> Subsystem/4(VISD_LaneC1L_rad)
  VLIC_EstLaneC1L_rad/1 -> Subsystem/5(VLIC_EstLaneC1L_rad)
  VISD_LaneC2L_rat/1 -> Subsystem/6(VISD_LaneC2L_rat)
  VLIC_EstLaneC2L_rat/1 -> Subsystem/7(VLIC_EstLaneC2L_rat)
  VISD_LaneC3L_rat/1 -> Subsystem/8(VISD_LaneC3L_rat)
  VLIC_EstLaneC3L_rat/1 -> Subsystem/9(VLIC_EstLaneC3L_rat)
  [VLIC_EstViewRangeEndL_m] -> Subsystem/11(VLIC_EstViewRangeEndL_m)
  [VISD_ViewRangeEndL_m] -> Subsystem/10(VISD_ViewRangeEndL_m)
  Subsystem/1(OptLaneC0L) -> Unit Delay1/1
  Subsystem/2(OptLaneC1L) -> Unit Delay2/1
  Subsystem/3(OptLaneC2L) -> Unit Delay3/1
  Subsystem/4(OptLaneC3L) -> Unit Delay4/1
  Subsystem/5(OptViewRange_L) -> Unit Delay5/1

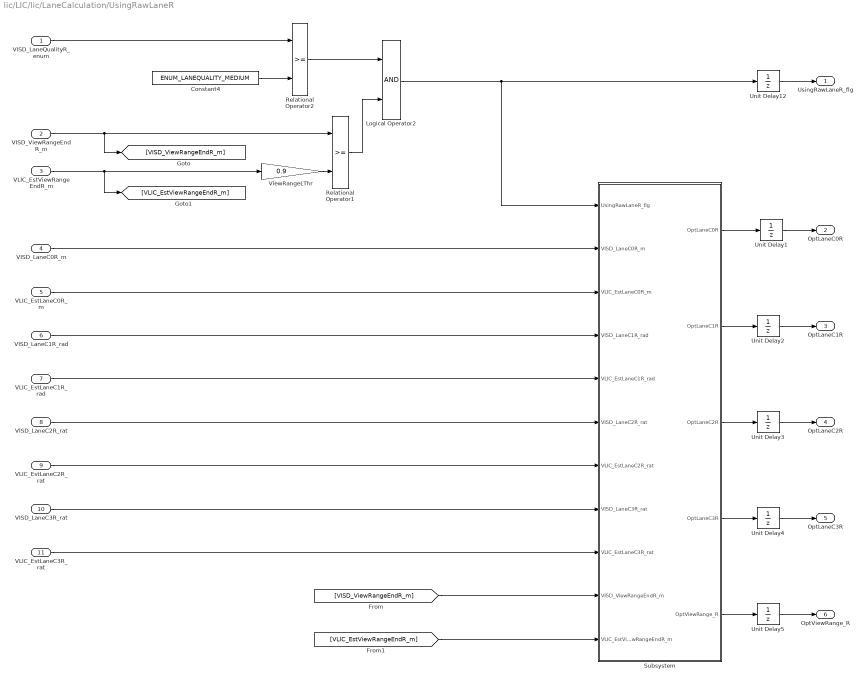
== system lic/LIC/lic/LaneCalculation/UsingRawLaneR ==
  VISD_LaneQualityR_enum : Inport
  VISD_ViewRangeEndR_m : Inport  Port=2
  VLIC_EstViewRangeEndR_m : Inport  Port=3
  VISD_LaneC0R_m : Inport  Port=4
  VLIC_EstLaneC0R_m : Inport  Port=5
  VISD_LaneC1R_rad : Inport  Port=6
  VLIC_EstLaneC1R_rad : Inport  Port=7
  VISD_LaneC2R_rat : Inport  Port=8
  VLIC_EstLaneC2R_rat : Inport  Port=9
  VISD_LaneC3R_rat : Inport  Port=10
  VLIC_EstLaneC3R_rat : Inport  Port=11
  Constant4 : Constant  Value=ENUM_LANEQUALITY_MEDIUM
  Logical Operator2 : Logic  AllPortsSameDT=off  OutDataTypeStr=boolean
  Relational Operator1 : RelationalOperator  OutDataTypeStr=boolean  RndMeth=Nearest
  Relational Operator2 : RelationalOperator  OutDataTypeStr=boolean  RndMeth=Nearest
  Subsystem : Subsystem
  Unit Delay{1..5,12} (6 alike) : UnitDelay  SampleTime=-1  HasFrameUpgradeWarning=on
  ViewRangeLThr : Gain  Gain=0.9
  UsingRawLaneR_flg : Outport
  OptLaneC0R : Outport  Port=2
  OptLaneC1R : Outport  Port=3
  OptLaneC2R : Outport  Port=4
  OptLaneC3R : Outport  Port=5
  OptViewRange_R : Outport  Port=6
  wires:
  Unit Delay5/1 -> OptViewRange_R/1
  Unit Delay4/1 -> OptLaneC3R/1
  Unit Delay3/1 -> OptLaneC2R/1
  Unit Delay2/1 -> OptLaneC1R/1
  Unit Delay1/1 -> OptLaneC0R/1
  Unit Delay12/1 -> UsingRawLaneR_flg/1
  Relational Operator1/1 -> Logical Operator2/2
  ViewRangeLThr/1 -> Relational Operator1/2
  VLIC_EstViewRangeEndR_m/1 -> [VLIC_EstViewRangeEndR_m], ViewRangeLThr/1
  VISD_ViewRangeEndR_m/1 -> [VISD_ViewRangeEndR_m], Relational Operator1/1
  Relational Operator2/1 -> Logical Operator2/1
  Constant4/1 -> Relational Operator2/2
  VISD_LaneQualityR_enum/1 -> Relational Operator2/1
  Logical Operator2/1 -> Subsystem/1(UsingRawLaneR_flg), Unit Delay12/1
  VISD_LaneC0R_m/1 -> Subsystem/2(VISD_LaneC0R_m)
  VLIC_EstLaneC0R_m/1 -> Subsystem/3(VLIC_EstLaneC0R_m)
  VISD_LaneC1R_rad/1 -> Subsystem/4(VISD_LaneC1R_rad)
  VLIC_EstLaneC1R_rad/1 -> Subsystem/5(VLIC_EstLaneC1R_rad)
  VISD_LaneC2R_rat/1 -> Subsystem/6(VISD_LaneC2R_rat)
  VLIC_EstLaneC2R_rat/1 -> Subsystem/7(VLIC_EstLaneC2R_rat)
  VISD_LaneC3R_rat/1 -> Subsystem/8(VISD_LaneC3R_rat)
  VLIC_EstLaneC3R_rat/1 -> Subsystem/9(VLIC_EstLaneC3R_rat)
  [VLIC_EstViewRangeEndR_m] -> Subsystem/11(VLIC_EstViewRangeEndR_m)
  [VISD_ViewRangeEndR_m] -> Subsystem/10(VISD_ViewRangeEndR_m)
  Subsystem/1(OptLaneC0R) -> Unit Delay1/1
  Subsystem/2(OptLaneC1R) -> Unit Delay2/1
  Subsystem/3(OptLaneC2R) -> Unit Delay3/1
  Subsystem/4(OptLaneC3R) -> Unit Delay4/1
  Subsystem/5(OptViewRange_R) -> Unit Delay5/1

== system lic/LIC/lic/LaneCalculation/Using_estimator_LeftLane ==
  VISD_LaneQualityL_enum : Inport
  VISD_ViewRangeEndL_m : Inport  Port=2
  VLIC_EstViewRangeEndL_m : Inport  Port=3
  Constant1 : Constant  Value=KLIC_LANEQUALITY_rat
  Constant2 : Constant  Value=KLIC_LANEQUALITYHysis_rat
  Constant6 : Constant  Value=ENUM_LANEQUALITY_MEDIUM
  Hysteresis : adcu_lib/Hysteresis  SystemSampleTime=-1  VariantActivationTime=update diagram  Latency=0  AutoFrameSizeCalculation=off
      settings: SourceProductName=ADAS Reusable Library
  Logical Operator4 : Logic  AllPortsSameDT=off  OutDataTypeStr=boolean
  Relational Operator5 : RelationalOperator  OutDataTypeStr=boolean  RndMeth=Nearest
  Relational Operator6 : RelationalOperator  OutDataTypeStr=boolean  RndMeth=Nearest
  ViewRangeL : Gain  Gain=0.5
  VLIC_LeftLaneAvail_flg : Outport
  wires:
  Relational Operator6/1 -> Logical Operator4/1
  Logical Operator4/1 -> VLIC_LeftLaneAvail_flg/1  "VLIC_LeftLaneAvail_flg"
  ViewRangeL/1 -> Relational Operator5/2
  Relational Operator5/1 -> Logical Operator4/2  "VRTiming_L"
  VLIC_EstViewRangeEndL_m/1 -> ViewRangeL/1
  VISD_LaneQualityL_enum/1 -> Relational Operator6/1
  Constant6/1 -> Relational Operator6/2
  VISD_ViewRangeEndL_m/1 -> Relational Operator5/1
  [VLIC_HLQualityL_rat] -> Hysteresis/1
  Constant1/1 -> Hysteresis/2
  Constant2/1 -> Hysteresis/3

== system lic/LIC/lic/LaneCalculation/Using_estimator_RightLane ==
  VISD_LaneQualityR_enum : Inport
  VISD_ViewRangeEndR_m : Inport  Port=2
  VLIC_EstViewRangeEndR_m : Inport  Port=3
  Constant7 : Constant  Value=ENUM_LANEQUALITY_MEDIUM
  Logical Operator5 : Logic  AllPortsSameDT=off  OutDataTypeStr=boolean
  Relational Operator7 : RelationalOperator  OutDataTypeStr=boolean  RndMeth=Nearest
  Relational Operator8 : RelationalOperator  OutDataTypeStr=boolean  RndMeth=Nearest
  ViewRangeR : Gain  Gain=0.5
  VLIC_RightLaneAvail_flg : Outport
  wires:
  VISD_ViewRangeEndR_m/1 -> Relational Operator7/1
  ViewRangeR/1 -> Relational Operator7/2
  VISD_LaneQualityR_enum/1 -> Relational Operator8/1
  Constant7/1 -> Relational Operator8/2
  VLIC_EstViewRangeEndR_m/1 -> ViewRangeR/1
  Relational Operator7/1 -> Logical Operator5/2  "VRTiming_R"
  Relational Operator8/1 -> Logical Operator5/1
  Logical Operator5/1 -> VLIC_RightLaneAvail_flg/1  "VLIC_RightLaneAvail_flg"

== system lic/LIC/lic/LaneInfo/Hysteresis_LessThan1 ==
  Input : Inport
  Switch_on_point : Inport  Port=2
  Switch_off_point : Inport  Port=3
  Logical Operator1 : Logic  AllPortsSameDT=off  OutDataTypeStr=boolean
  Logical Operator2 : Logic  Operator=NOT  AllPortsSameDT=off  OutDataTypeStr=boolean
  Logical Operator3 : Logic  Operator=OR  AllPortsSameDT=off  OutDataTypeStr=boolean
  Relational Operator : RelationalOperator  Operator=<=  OutDataTypeStr=boolean  RndMeth=Nearest
  Relational Operator1 : RelationalOperator  OutDataTypeStr=boolean  RndMeth=Nearest
  Unit Delay : UnitDelay  SampleTime=-1  HasFrameUpgradeWarning=on
  Output : Outport
  wires:
  Switch_on_point/1 -> Relational Operator/2
  Switch_off_point/1 -> Relational Operator1/2
  Logical Operator2/1 -> Logical Operator1/2
  Unit Delay/1 -> Logical Operator3/1
  Input/1 -> Relational Operator/1, Relational Operator1/1
  Relational Operator/1 -> Logical Operator3/2
  Logical Operator3/1 -> Logical Operator1/1
  Relational Operator1/1 -> Logical Operator2/1
  Logical Operator1/1 -> Output/1, Unit Delay/1

== system lic/LIC/lic/LaneInfo/SR-Latch1 ==
  set : Inport
  reset : Inport  Port=2
  Logical Operator : Logic  AllPortsSameDT=off  OutDataTypeStr=boolean
  Logical Operator1 : Logic  Operator=NOT  AllPortsSameDT=off  OutDataTypeStr=boolean
  Switch1 : Switch  Criteria=u2 ~= 0  Threshold=0.5
      settings: AttributesFormatString=<Criteria=%<Criteria>>
  Switch2 : Switch  Criteria=u2 ~= 0  Threshold=0.5
      settings: AttributesFormatString=<Criteria=%<Criteria>>
  Unit Delay : UnitDelay  SampleTime=-1  HasFrameUpgradeWarning=on
  latched : Outport
  wires:
  Logical Operator1/1 -> Switch2/1, Logical Operator/2
  Logical Operator/1 -> Switch1/2
  Switch2/1 -> Switch1/3
  Unit Delay/1 -> Switch2/3
  reset/1 -> Logical Operator1/1, Switch2/2
  set/1 -> Logical Operator/1, Switch1/1
  Switch1/1 -> latched/1, Unit Delay/1

== system lic/LIC/lic/LaneInfo/Timer1 ==
  Enable : EnablePort  StatesWhenEnabling=reset  ZeroCross=off
  Constant : Constant  Value=C_TICK_TIME_S
  Sum : Sum  Inputs=|++  InputSameDT=on  SaturateOnIntegerOverflow=on
  Unit Delay : UnitDelay  SampleTime=-1  HasFrameUpgradeWarning=on
  Timer (sec) : Outport  OutputWhenDisabled=reset  InitialOutput=0
  wires:
  Constant/1 -> Sum/1
  Sum/1 -> Unit Delay/1
  Unit Delay/1 -> Sum/2, Timer (sec)/1

== system lic/LIC/lic/LaneInfo/Timer2 ==
  Enable : EnablePort  StatesWhenEnabling=reset  ZeroCross=off
  Constant : Constant  Value=C_TICK_TIME_S
  Sum : Sum  Inputs=|++  InputSameDT=on  SaturateOnIntegerOverflow=on
  Unit Delay : UnitDelay  SampleTime=-1  HasFrameUpgradeWarning=on
  Timer (sec) : Outport  OutputWhenDisabled=reset  InitialOutput=0
  wires:
  Unit Delay/1 -> Timer (sec)/1, Sum/2
  Sum/1 -> Unit Delay/1
  Constant/1 -> Sum/1

== system lic/LIC/lic/LaneInfo/Timer3 ==
  Enable : EnablePort  StatesWhenEnabling=reset  ZeroCross=off
  Constant : Constant  Value=C_TICK_TIME_S
  Sum : Sum  Inputs=|++  InputSameDT=on  SaturateOnIntegerOverflow=on
  Unit Delay : UnitDelay  SampleTime=-1  HasFrameUpgradeWarning=on
  Timer (sec) : Outport  OutputWhenDisabled=reset  InitialOutput=0
  wires:
  Unit Delay/1 -> Timer (sec)/1, Sum/2
  Sum/1 -> Unit Delay/1
  Constant/1 -> Sum/1

== system lic/LIC/lic/LaneInfo/Timer4 ==
  Enable : EnablePort  StatesWhenEnabling=reset  ZeroCross=off
  Constant : Constant  Value=C_TICK_TIME_S
  Sum : Sum  Inputs=|++  InputSameDT=on  SaturateOnIntegerOverflow=on
  Unit Delay : UnitDelay  SampleTime=-1  HasFrameUpgradeWarning=on
  Timer (sec) : Outport  OutputWhenDisabled=reset  InitialOutput=0
  wires:
  Unit Delay/1 -> Timer (sec)/1, Sum/2
  Sum/1 -> Unit Delay/1
  Constant/1 -> Sum/1

== system lic/LIC/lic/LaneInfo/Timer5 ==
  Enable : EnablePort  StatesWhenEnabling=reset  ZeroCross=off
  Constant : Constant  Value=C_TICK_TIME_S
  Sum : Sum  Inputs=|++  InputSameDT=on  SaturateOnIntegerOverflow=on
  Unit Delay : UnitDelay  SampleTime=-1  HasFrameUpgradeWarning=on
  Timer (sec) : Outport  OutputWhenDisabled=reset  InitialOutput=0
  wires:
  Constant/1 -> Sum/1
  Sum/1 -> Unit Delay/1
  Unit Delay/1 -> Sum/2, Timer (sec)/1

== system lic/LIC/lic/LaneInfo/Timer7 ==
  Enable : EnablePort  StatesWhenEnabling=reset  ZeroCross=off
  Constant : Constant  Value=C_TICK_TIME_S
  Sum : Sum  Inputs=|++  InputSameDT=on  SaturateOnIntegerOverflow=on
  Unit Delay : UnitDelay  SampleTime=-1  HasFrameUpgradeWarning=on
  Timer (sec) : Outport  OutputWhenDisabled=reset  InitialOutput=0
  wires:
  Constant/1 -> Sum/1
  Sum/1 -> Unit Delay/1
  Unit Delay/1 -> Sum/2, Timer (sec)/1

== system lic/LIC/lic/LaneInfo/divide1 ==
  dividend : Inport
  divisor : Inport  Port=2
  default_value : Inport  Port=3
  Divide : Product  Inputs=*/
  Interval Test : simulink/Logic and Bit Operations/Interval Test  IntervalClosedRight=on  uplimit=0.00001  IntervalClosedLeft=on  lowlimit=-0.00001  OutDataTypeStr=boolean
  Logical Operator : Logic  Operator=NOT  Inputs=1  AllPortsSameDT=off  OutDataTypeStr=boolean
  Switch : Switch  Criteria=u2 ~= 0  Threshold=0.5
  quotient : Outport
  wires:
  Logical Operator/1 -> Switch/2
  default_value/1 -> Switch/3  "default_value"
  Interval Test/1 -> Logical Operator/1
  Switch/1 -> quotient/1
  Divide/1 -> Switch/1
  divisor/1 -> Interval Test/1, Divide/2  "divisor"
  dividend/1 -> Divide/1  "dividend"

== system lic/LIC/lic/LaneInfo/rad2deg1 ==
  u : Inport
  Gain : Gain  Gain=180/pi
  y : Outport
  wires:
  u/1 -> Gain/1  "u"
  Gain/1 -> y/1  "y"

== system lic/LIC/lic/LaneCalculation/C1L_Bias/Forgetting_factor ==
  C1LBias_new : Inport
  Enable : EnablePort
  FF : Stateflow chart  TreatAsAtomicUnit=on
  Forget_factor : Constant  Value=0.99933  OutDataTypeStr=single
  Terminator : Terminator
  C1L_Bias : Outport
  wires:
  C1LBias_new/1 -> FF/1(C1LBias_new)
  FF/1(C1L_Bias) -> C1L_Bias/1
  FF/2(P_L) -> Terminator/1
  Forget_factor/1 -> FF/2(Forget_Factor)

== system lic/LIC/lic/LaneCalculation/C1R_Bias/Forgetting_factor ==
  C1RBias_new : Inport
  Enable : EnablePort
  FF : Stateflow chart  TreatAsAtomicUnit=on
  Forget_factor : Constant  Value=0.99933  OutDataTypeStr=single
  Terminator : Terminator
  C1R_Bias : Outport
  wires:
  C1RBias_new/1 -> FF/1(C1RBias_new)
  FF/1(C1R_Bias) -> C1R_Bias/1
  FF/2(P_R) -> Terminator/1
  Forget_factor/1 -> FF/2(Forget_Factor)

== system lic/LIC/lic/LaneCalculation/C1R_Bias/divide1 ==
  dividend : Inport
  divisor : Inport  Port=2
  default_value : Inport  Port=3
  Divide : Product  Inputs=*/
  Interval Test : simulink/Logic and Bit Operations/Interval Test  IntervalClosedRight=on  uplimit=0.00001  IntervalClosedLeft=on  lowlimit=-0.00001  OutDataTypeStr=boolean
  Logical Operator : Logic  Operator=NOT  Inputs=1  AllPortsSameDT=off  OutDataTypeStr=boolean
  Switch : Switch  Criteria=u2 ~= 0  Threshold=0.5
  quotient : Outport
  wires:
  dividend/1 -> Divide/1  "dividend"
  divisor/1 -> Divide/2, Interval Test/1  "divisor"
  Divide/1 -> Switch/1
  Switch/1 -> quotient/1
  Interval Test/1 -> Logical Operator/1
  default_value/1 -> Switch/3  "default_value"
  Logical Operator/1 -> Switch/2

== system lic/LIC/lic/LaneCalculation/C1R_Bias/divide4 ==
  dividend : Inport
  divisor : Inport  Port=2
  default_value : Inport  Port=3
  Divide : Product  Inputs=*/
  Interval Test : simulink/Logic and Bit Operations/Interval Test  IntervalClosedRight=on  uplimit=0.00001  IntervalClosedLeft=on  lowlimit=-0.00001  OutDataTypeStr=boolean
  Logical Operator : Logic  Operator=NOT  Inputs=1  AllPortsSameDT=off  OutDataTypeStr=boolean
  Switch : Switch  Criteria=u2 ~= 0  Threshold=0.5
  quotient : Outport
  wires:
  Logical Operator/1 -> Switch/2
  default_value/1 -> Switch/3  "default_value"
  Interval Test/1 -> Logical Operator/1
  Switch/1 -> quotient/1
  Divide/1 -> Switch/1
  divisor/1 -> Interval Test/1, Divide/2  "divisor"
  dividend/1 -> Divide/1  "dividend"

== system lic/LIC/lic/LaneCalculation/LaneResidual_Calculation/divide1 ==
  dividend : Inport
  divisor : Inport  Port=2
  default_value : Inport  Port=3
  Divide : Product  Inputs=*/
  Interval Test : simulink/Logic and Bit Operations/Interval Test  IntervalClosedRight=on  uplimit=0.00001  IntervalClosedLeft=on  lowlimit=-0.00001  OutDataTypeStr=boolean
  Logical Operator : Logic  Operator=NOT  Inputs=1  AllPortsSameDT=off  OutDataTypeStr=boolean
  Switch : Switch  Criteria=u2 ~= 0  Threshold=0.5
  quotient : Outport
  wires:
  Logical Operator/1 -> Switch/2
  default_value/1 -> Switch/3  "default_value"
  Interval Test/1 -> Logical Operator/1
  Switch/1 -> quotient/1
  Divide/1 -> Switch/1
  divisor/1 -> Interval Test/1, Divide/2  "divisor"
  dividend/1 -> Divide/1  "dividend"

== system lic/LIC/lic/LaneCalculation/LaneResidual_Calculation/divide3 ==
  dividend : Inport
  divisor : Inport  Port=2
  default_value : Inport  Port=3
  Divide : Product  Inputs=*/
  Interval Test : simulink/Logic and Bit Operations/Interval Test  IntervalClosedRight=on  uplimit=0.00001  IntervalClosedLeft=on  lowlimit=-0.00001  OutDataTypeStr=boolean
  Logical Operator : Logic  Operator=NOT  Inputs=1  AllPortsSameDT=off  OutDataTypeStr=boolean
  Switch : Switch  Criteria=u2 ~= 0  Threshold=0.5
  quotient : Outport
  wires:
  dividend/1 -> Divide/1  "dividend"
  divisor/1 -> Divide/2, Interval Test/1  "divisor"
  Divide/1 -> Switch/1
  Switch/1 -> quotient/1
  Interval Test/1 -> Logical Operator/1
  default_value/1 -> Switch/3  "default_value"
  Logical Operator/1 -> Switch/2

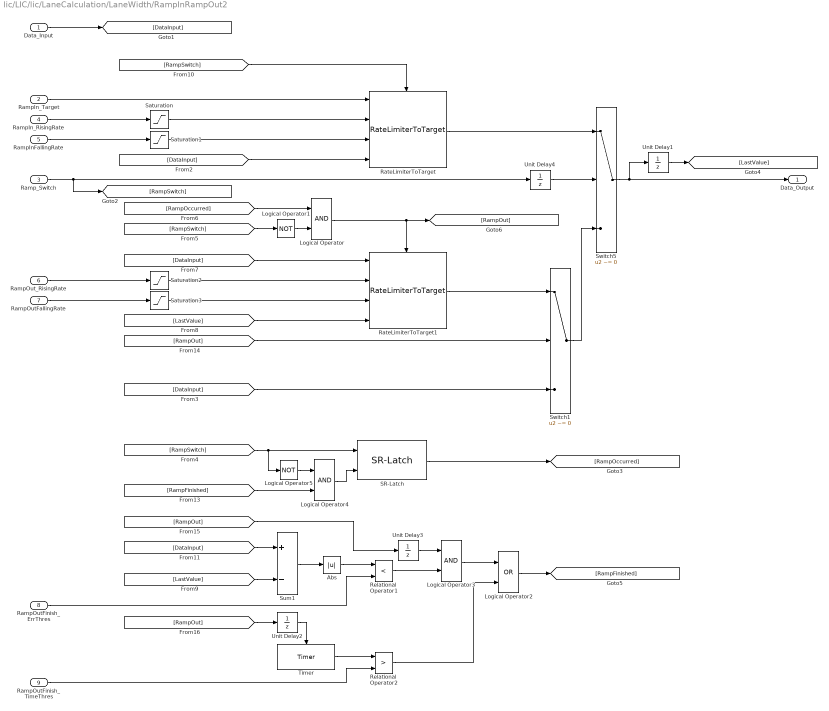
== system lic/LIC/lic/LaneCalculation/LaneWidth/RampInRampOut2 ==
  Data_Input : Inport
  RampIn_Target : Inport  Port=2
  Ramp_Switch : Inport  Port=3
  RampIn_RisingRate : Inport  Port=4
  RampInFallingRate : Inport  Port=5
  RampOut_RisingRate : Inport  Port=6
  RampOutFallingRate : Inport  Port=7
  RampOutFinish_ErrThres : Inport  Port=8
  RampOutFinish_TimeThres : Inport  Port=9
  Abs : Abs
  Logical Operator : Logic  AllPortsSameDT=off  OutDataTypeStr=boolean
  Logical Operator1 : Logic  Operator=NOT  AllPortsSameDT=off  OutDataTypeStr=boolean
  Logical Operator2 : Logic  Operator=OR  AllPortsSameDT=off  OutDataTypeStr=boolean
  Logical Operator3 : Logic  AllPortsSameDT=off  OutDataTypeStr=boolean
  Logical Operator4 : Logic  AllPortsSameDT=off  OutDataTypeStr=boolean
  Logical Operator5 : Logic  Operator=NOT  AllPortsSameDT=off  OutDataTypeStr=boolean
  RateLimiterToTarget : adcu_lib/RateLimiterToTarget  SystemSampleTime=-1  VariantActivationTime=update diagram  Latency=0  AutoFrameSizeCalculation=off
      settings: SourceProductName=ADAS Reusable Library
  RateLimiterToTarget1 : adcu_lib/RateLimiterToTarget  SystemSampleTime=-1  VariantActivationTime=update diagram  Latency=0  AutoFrameSizeCalculation=off
      settings: SourceProductName=ADAS Reusable Library
  Relational Operator1 : RelationalOperator  Operator=<  OutDataTypeStr=boolean  RndMeth=Nearest
  Relational Operator2 : RelationalOperator  Operator=>  OutDataTypeStr=boolean  RndMeth=Nearest
  SR-Latch : adcu_lib/SR-Latch  SystemSampleTime=-1  VariantActivationTime=update diagram  Latency=0  AutoFrameSizeCalculation=off
      settings: SourceProductName=ADAS Reusable Library
  Saturation : Saturate  UpperLimit=inf  LowerLimit=0
  Saturation1 : Saturate  UpperLimit=0  LowerLimit=-inf
  Saturation2 : Saturate  UpperLimit=inf  LowerLimit=0
  Saturation3 : Saturate  UpperLimit=0  LowerLimit=-inf
  Sum1 : Sum  Inputs=+-
  Switch1 : Switch  Criteria=u2 ~= 0
  Switch5 : Switch  Criteria=u2 ~= 0
  Timer : adcu_lib/Timer  SystemSampleTime=-1  VariantActivationTime=update diagram  Latency=0  AutoFrameSizeCalculation=off
      settings: SourceProductName=ADAS Reusable Library
  Unit Delay{1..4} (4 alike) : UnitDelay  SampleTime=-1  HasFrameUpgradeWarning=on
  Data_Output : Outport  InitialOutput=[0]
  wires:
  Data_Input/1 -> [DataInput]
  RateLimiterToTarget/1 -> Switch5/1
  [RampSwitch] -> RateLimiterToTarget/Enable
  RampIn_Target/1 -> RateLimiterToTarget/1
  RampIn_RisingRate/1 -> Saturation/1
  RampInFallingRate/1 -> Saturation1/1
  [DataInput] -> RateLimiterToTarget/4
  [DataInput] -> Switch1/3
  Switch5/1 -> Unit Delay1/1, Data_Output/1
  [RampSwitch] -> SR-Latch/1, Logical Operator5/1
  SR-Latch/1 -> [RampOccurred]
  Switch1/1 -> Switch5/3
  [RampSwitch] -> Logical Operator1/1
  [RampOccurred] -> Logical Operator/1
  Logical Operator1/1 -> Logical Operator/2
  [DataInput] -> RateLimiterToTarget1/1
  RampOut_RisingRate/1 -> Saturation2/1
  RampOutFallingRate/1 -> Saturation3/1
  [LastValue] -> RateLimiterToTarget1/4
  Unit Delay1/1 -> [LastValue]
  [DataInput] -> Sum1/1
  [LastValue] -> Sum1/2
  Sum1/1 -> Abs/1
  Abs/1 -> Relational Operator1/1
  RampOutFinish_ErrThres/1 -> Relational Operator1/2
  [RampOut] -> Unit Delay2/1
  Timer/1 -> Relational Operator2/1
  RampOutFinish_TimeThres/1 -> Relational Operator2/2
  Relational Operator1/1 -> Logical Operator3/2
  Relational Operator2/1 -> Logical Operator2/2
  Logical Operator2/1 -> [RampFinished]
  [RampFinished] -> Logical Operator4/2
  Unit Delay2/1 -> Timer/Enable
  Logical Operator3/1 -> Logical Operator2/1
  Logical Operator5/1 -> Logical Operator4/1
  Logical Operator4/1 -> SR-Latch/2
  Logical Operator/1 -> RateLimiterToTarget1/Enable, [RampOut]
  Ramp_Switch/1 -> Unit Delay4/1, [RampSwitch]
  RateLimiterToTarget1/1 -> Switch1/1
  Unit Delay4/1 -> Switch5/2
  [RampOut] -> Switch1/2
  Unit Delay3/1 -> Logical Operator3/1
  [RampOut] -> Unit Delay3/1
  Saturation/1 -> RateLimiterToTarget/2
  Saturation1/1 -> RateLimiterToTarget/3
  Saturation3/1 -> RateLimiterToTarget1/3
  Saturation2/1 -> RateLimiterToTarget1/2

== system lic/LIC/lic/LaneCalculation/LaneWidth/Timer2 ==
  Enable : EnablePort  StatesWhenEnabling=reset  ZeroCross=off
  Constant : Constant  Value=C_TICK_TIME_S
  Sum : Sum  Inputs=|++  InputSameDT=on  SaturateOnIntegerOverflow=on
  Unit Delay : UnitDelay  SampleTime=-1  HasFrameUpgradeWarning=on
  Timer (sec) : Outport  OutputWhenDisabled=reset  InitialOutput=0
  wires:
  Unit Delay/1 -> Timer (sec)/1, Sum/2
  Sum/1 -> Unit Delay/1
  Constant/1 -> Sum/1
